simulink model "power_spec"  (R2019a)
settings: Solver=VariableStepAuto  StartTime=0.0  StopTime=10.0  RelTol=1e-3
InitFcn:
  | M=4;
  | Fs=10e6;
  | Fb=log2(M)*Fs;
  | 
  | PT=5.0;
  | A=1/100;
  | PR=A*PT;
  | 
  | P=[0,-2,-3];
  | T=[0,15,50]*10^(-9);
  | fd=70;
undefined symbols (not defined in the file or in its folder): doppler
libraries: commrandsrc3 x1, commdigbbndam3 x1, commchan3 x1
settings Model: Creator=charles  LastModifiedBy=charles

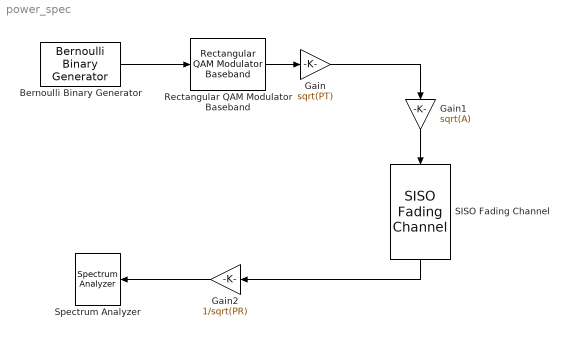
== system power_spec ==
  Bernoulli Binary Generator : commrandsrc3/Bernoulli Binary Generator  ProbabilityOfZero=0.5  SeedSource=Parameter  Seed=61  SampleTime=1/Fb  SamplesPerFrame=log2(M)  OutputDataType=single  SimulateUsing=Interpreted execution
      settings: SourceProductName=Communications Toolbox
  Gain : Gain  Gain=sqrt(PT)
  Gain1 : Gain  Gain=sqrt(A)
  Gain2 : Gain  Gain=1/sqrt(PR)
  Rectangular QAM Modulator Baseband : commdigbbndam3/Rectangular QAM Modulator Baseband  M=M  InType=Bit  Enc=Gray  Mapping=[0:15]  PowType=Average Power  MinDist=2  AvgPow=1  PeakPow=1  Ph=0  outDtype=double  outWordLen=16  outUDDataType=sfix(16)  outFracLenMode=Best precision  outFracLen=15  outDataTypeStr=double  outLastDataTypeStr=double
      settings: SourceProductName=Communications Toolbox
  SISO Fading Channel : commchan3/SISO Fading Channel  InheritSampleRate=on  SampleRate=1  PathDelays=T  AveragePathGains=P  NormalizePathGains=on  FadingDistribution=Rayleigh  KFactor=3  DirectPathDopplerShift=0  DirectPathInitialPhase=0  MaximumDopplerShift=fd  DopplerSpectrum=doppler('Jakes')  ChannelInterpolationMethod=Polyphase  RandomStream=mt19937ar with seed  RandomNumGenerator=mt19937ar  Seed=73  PathGainsOutputPort=off  ChannelFilterDelayOutputPort=off  SimulateUsing=Interpreted execution  Visualization=Off  PathsForDopplerDisplay=1  SamplesToDisplay=25%
      settings: SourceProductName=Communications Toolbox
  Spectrum Analyzer : SpectrumAnalyzer
  wires:
  Bernoulli Binary Generator/1 -> Rectangular QAM Modulator Baseband/1
  Rectangular QAM Modulator Baseband/1 -> Gain/1
  Gain1/1 -> SISO Fading Channel/1
  Gain/1 -> Gain1/1
  SISO Fading Channel/1 -> Gain2/1
  Gain2/1 -> Spectrum Analyzer/1
